simulink model "P_2_1_k_Csillapitott_inga"  (R2021b)
settings: Solver=VariableStepAuto  StartTime=0.0  StopTime=10.0  MaxStep=0.01  RelTol=1e-3
settings Model: Creator=davidpaksi  LastModifiedBy=davidpaksi

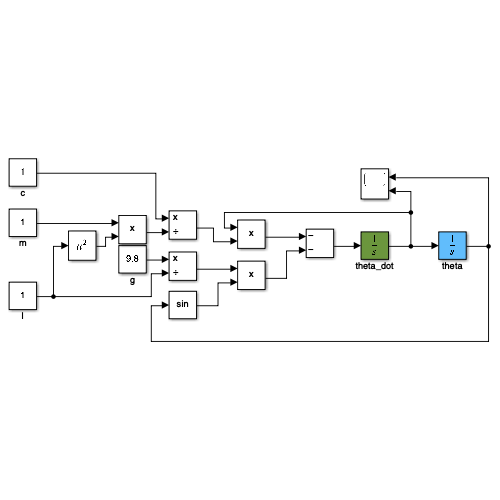
[thumbnail: Simulink's stored preview of the top-level diagram]
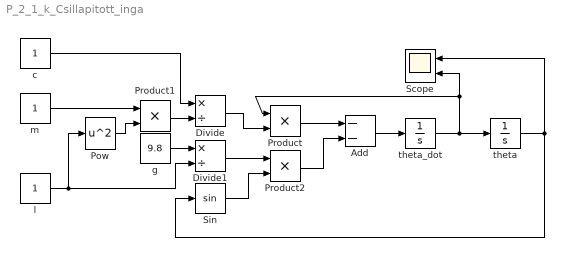
== system P_2_1_k_Csillapitott_inga ==
  Add : Sum  Inputs=--
  Divide : Product  Inputs=*/
  Divide1 : Product  Inputs=*/
  Pow : Math  Operator=square  SignedPower=on  RndMeth=Zero  SaturateOnIntegerOverflow=on
  Product : Product
  Product1 : Product
  Product2 : Product
  Scope : Scope  NumInputPorts=2
  Sin : Trigonometry
  c : Constant
  g : Constant  Value=9.8
  l : Constant
  m : Constant
  theta : Integrator  InitialCondition=1
  theta_dot : Integrator
  wires:
  theta_dot/1 -> Product/1, Scope/2, theta/1
  Add/1 -> theta_dot/1
  Product/1 -> Add/1
  c/1 -> Divide/1
  Product1/1 -> Divide/2
  m/1 -> Product1/1
  Pow/1 -> Product1/2
  l/1 -> Divide1/2, Pow/1
  Divide/1 -> Product/2
  Product2/1 -> Add/2
  Divide1/1 -> Product2/1
  g/1 -> Divide1/1
  Sin/1 -> Product2/2
  theta/1 -> Sin/1, Scope/1
